simulink model "Converter_3"  (R2018a)
settings: Solver=ode45  StartTime=0.0  StopTime=3  RelTol=1e-3
InitFcn:
  | Ts=4e-4;
  | Ts_Power=Ts;
  | Ts_Control=Ts;
  | P_order = 0.9;
  | Q_order= 0.4;
  | V_order=1;
  | w_order = 1;
  | 
  | %outer loop
  | Kpvd=1;
  | Kivd=400;
  | Kpvq=1;
  | Kivq=10;
  | 
  | %inner loop
  | Kp=0.3;
  | Ki=5;
  | 
  | %Droop;
  | m=0.2;
  | n=0.1;
  | 
  | 
  | 
  | X=0.15;
  | wb=2*pi*60;
  | Sb=10e3; %2*Num MW
  | Vb=260;
  | Vconv=260;
  | Zb=Vb^2/Sb;
  | 
  | 
  | %% Tirp Transmision line
  | Tstep3=20; % trip line: Xg_start-->Xg_mid
  | Tstep2=30; % trip line: Xg_mid-->Xg_final
  | 
  | 
  | 
  | Xg_start=1.19; Xg_mid=1.2; Xg_final=1.21;
  | 
  | 
  | Xgpu2=Xg_mid*Xg_final/(Xg_final-Xg_mid);
  | Xgpu3=Xg_start*(Xg_final*Xgpu2)/(Xg_final*Xgpu2-Xg_start*(Xg_final+Xgpu2));
  | 
  | %Line 1
  | Xgpu1=Xg_final;
  | Rgpu1=0.1*Xgpu1;%Rg=0.1*Xg;
  | Xg1=Xgpu1*Zb;
  | Lg1=Xg1/wb;   %H
  | Rg1=Rgpu1*Zb; %ohm
  | %Line 2
  | Rgpu2=0.1*Xgpu2;%Rg=0.1*Xg;
  | Xg2=Xgpu2*Zb;
  | Lg2=Xg2/wb;   %H
  | Rg2=Rgpu2*Zb; %ohm
  | %Line 3
  | Rgpu3=0.1*Xgpu3;%Rg=0.1*Xg;
  | Xg3=Xgpu3*Zb;
  | Lg3=Xg3/wb;   %H
  | Rg3=Rgpu3*Zb; %ohm
undefined symbols (not defined in the file or in its folder): DiscIntNeverNeededParam
libraries: powerlib x14, simulink x3, powerlib_meascontrol x2, powerlib_extras x1
Description:
  | Copyright 2008-2018 The MathWorks, Inc.
settings Model: Creator=MathWorks  LastModifiedBy=almut
settings DataIOCC: FinalStateName=xFinal2  LimitDataPoints=on  SaveFinalState=on  SaveFormat=Array  SignalLoggingSaveFormat=ModelDataLogs
settings OptimizationCC: ExpressionDepthLimit=2147483647  LifeSpan=inf
settings DebuggingCC: AlgebraicLoopMsg=none  UnderspecifiedInitializationDetection=Classic  MergeDetectMultiDrivingBlocksExec=none  SolverPrmCheckMsg=warning  FcnCallInpInsideContextMsg=warning  StateNameClashWarn=warning  SFUnexpectedBacktrackingDiag=warning  SFNoUnconditionalDefaultTransitionDiag=warning  SFExecutionAtInitializationDiag=none
settings HardwareCC: ProdBitPerPointer=32  ProdBitPerSizeT=32  ProdBitPerPtrDiffT=32  ProdLargestAtomicFloat=None  ProdIntDivRoundTo=Undefined  ProdEndianess=Unspecified  ProdWordSize=32  ProdHWDeviceType=32-bit Generic
settings ModelReferenceCC: PropagateSignalLabelsOutOfModel=off
settings CodeAppCC: StateflowObjectComments=on
settings GRTTargetCC: TargetLangStandard=C89/C90 (ANSI)  GeneratePreprocessorConditionals=Disable all  CombineOutputUpdateFcns=off  GRTInterface=on
settings ConfigComp: CovMetricSettings=dw  CovHtmlReporting=on  CovSaveCumulativeToWorkspaceVar=on  CovSaveSingleToWorkspaceVar=on  CovExternalEMLEnable=off  CovSFcnEnable=off
settings SimscapeCC: SimscapeNormalizeSystem=off

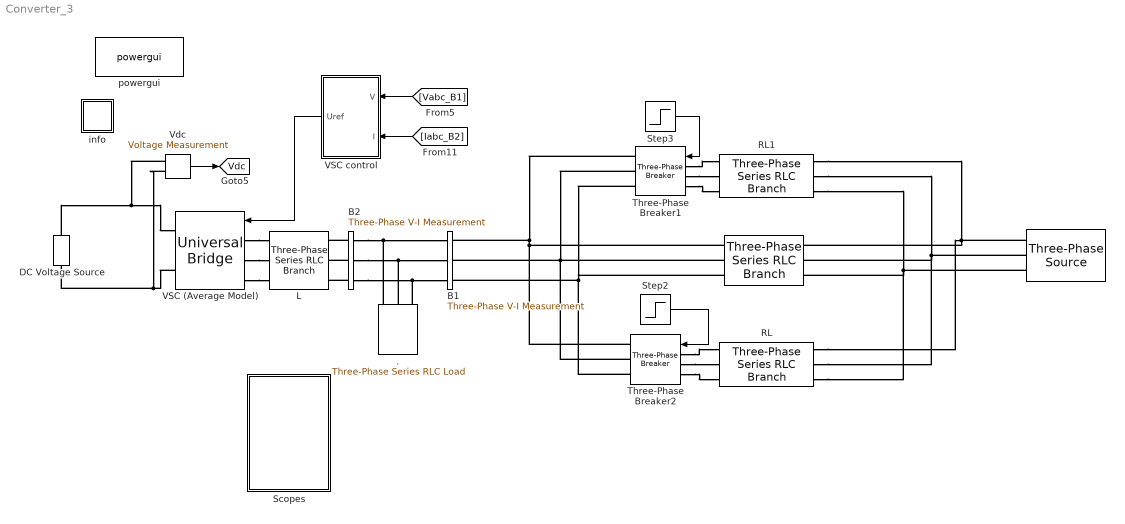
== system Converter_3 ==
  " " : powerlib/Elements/Three-Phase Series RLC Branch  LConnTagsString=A|B|C  RConnTagsString=A|B|C  BranchType=RL  Resistance=Rg1  Inductance=Lg1  Capacitance=[]  Measurements=None
  "   " : powerlib/Electrical Sources/Three-Phase Source  InternalConnection=Yg  VoltagePhases=off  Voltage=260  PhaseAngle=0  Voltage_phases=[25e3 25e3 25e3]/sqrt(3)  PhaseAngles_phases=[0 -120 +120]  Frequency=60  NonIdealSource=off  SpecifyImpedance=on  Resistance=0.8929  Inductance=16.58e-3  ShortCircuitLevel=2500e6  BaseVoltage=120e3  XRratio=7  BusType=swing  Pref=0  Qref=0  Prefabc=[10e3, 10e3, 10e3]  Qrefabc=[0, 0, 0]  Qmin=-inf  Qmax=inf
  "  ." : powerlib/Elements/Three-Phase Series RLC Load  LConnTagsString=A|B|C  Configuration=Y (grounded)  NominalVoltage=260  Vabc=[1e3 1e3 1e3]  Vabcp=[1e3 1e3 1e3]  NominalFrequency=60  UnbalancedPower=off  ActivePower=0  InductivePower=0  CapacitivePower=10e3*0.25  Pabc=[10e3 9e3 11e3]  QLabc=[100 90 110]  QCabc=[100 90 110]  Pabcp=[10e3 9e3 11e3]  QLabcp=[100 90 110]  QCabcp=[100 90 110]  Measurements=None  LoadType=constant Z
  B1 : powerlib/Measurements/Three-Phase V-I Measurement  VoltageMeasurement=phase-to-ground  SetLabelV=on  LabelV=Vabc_B1  Vpu=on  VpuLL=off  CurrentMeasurement=yes  SetLabelI=on  LabelI=Iabc_B1  Ipu=on  Pbase=10e3  Vbase=260  OutputType=Magnitude  PhasorSimulation=off  PSBequivalent=0
  B2 : powerlib/Measurements/Three-Phase V-I Measurement  VoltageMeasurement=phase-to-ground  SetLabelV=on  LabelV=Vabc_c  Vpu=on  VpuLL=off  CurrentMeasurement=yes  SetLabelI=on  LabelI=Iabc_B2  Ipu=on  Pbase=10e3  Vbase=260  OutputType=Magnitude  PhasorSimulation=off  PSBequivalent=0
  DC Voltage Source : powerlib/Electrical Sources/DC Voltage Source  Amplitude=500  Measurements=None
  L : powerlib/Elements/Three-Phase Series RLC Branch  LConnTagsString=A|B|C  RConnTagsString=A|B|C  BranchType=RL  Resistance=X/50*260^2/10e3  Inductance=X/(2*pi*60)*260^2/10e3  Capacitance=inf  Measurements=None
  RL : powerlib/Elements/Three-Phase Series RLC Branch  LConnTagsString=A|B|C  RConnTagsString=A|B|C  BranchType=RL  Resistance=Rg2  Inductance=Lg2  Capacitance=[]  Measurements=None
  RL1 : powerlib/Elements/Three-Phase Series RLC Branch  LConnTagsString=A|B|C  RConnTagsString=A|B|C  BranchType=RL  Resistance=Rg3  Inductance=Lg3  Capacitance=[]  Measurements=None
  Scopes : Subsystem
  Step2 : Step  Time=Tstep2  Before=1  After=0  SampleTime=0
  Step3 : Step  Time=Tstep3  Before=1  After=0  SampleTime=0
  Three-Phase Breaker1 : powerlib/Elements/Three-Phase Breaker  InitialState=closed  SwitchA=on  SwitchB=on  SwitchC=on  SwitchTimes=[1 1000]  External=on  BreakerResistance=0.001  SnubberResistance=1e6  SnubberCapacitance=inf  Measurements=None
  Three-Phase Breaker2 : powerlib/Elements/Three-Phase Breaker  InitialState=closed  SwitchA=on  SwitchB=on  SwitchC=on  SwitchTimes=[1 1000]  External=on  BreakerResistance=0.001  SnubberResistance=1e6  SnubberCapacitance=inf  Measurements=None
  VSC (Average Model) : powerlib/Power Electronics/Universal Bridge  Arms=3  SnubberResistance=1e5  SnubberCapacitance=inf  Device=Average-model based VSC  Ron=1e-3  Lon=0  ForwardVoltages="[  0  0  ]"  ForwardVoltage=0  GTOparameters=[ 10e-6 , 20e-6 ]  IGBTparameters=[ 1e-6 , 2e-6 ]  Measurements=None  Measurements_2=None  converterType=Rectifier
  VSC control : Subsystem
  "Vdc " : powerlib/Measurements/Voltage Measurement  Tag=PoWeRsYsTeMmEaSuReMeNt  PhasorSimulation=off  OutputType=Magnitude  PSBequivalent=0
  info : Subsystem
      settings: OpenFcn=showdemo(bdroot(gcb))
      mask Display: disp('?')
  powergui : powerlib/powergui  Priority=1  SimulationMode=Discrete  SampleTime=Ts_Power  frequency=60  Iterations=50  frequencyindice=0  Pbase=100e6  ErrMax=1e-4  UnitsV=kV  UnitsW=MW  buscounter=0  FunctionMessages=off  echomessages=off  EnableUseOfTLC=off  CurrentSourceSwitches=off  DisableSnubberDevices=off  DisableRonSwitches=off  DisableVfSwitches=off  DisplayEquations=off  SolverType=Tustin/Backward Euler (TBE)  Interpol=off  ExternalGateDelay=off  methode=off  Ts=100  x0status=blocks  SPID=off  SwTol=0  HookPort=off  RestoreLinks=warning  ResistiveCurrentMeasurement=off  Frange=[0:2:500]  Ylog=off  Xlog=on  ShowGrid=off  save=off  variable=ZData  structure=y1  ZoomFFT=off  StartTime=3  cycles=60  DisplayStyle=2  fundamental=60  FreqAxis=off  MaxFrequency=100  frequencyindicesteady=1  RmsSteady=1  display=off
  tag scope: Vdc=global
  wires:
  "Vdc "/1 -> [Vdc]
  [Vabc_B1] -> VSC control/1(V)
  [Iabc_B2] -> VSC control/2(I)
  VSC control/1(Uref) -> VSC (Average Model)/1
  Step2/1 -> Three-Phase Breaker2/1
  Step3/1 -> Three-Phase Breaker1/1
  connections:
  VSC (Average Model)/LConn1 -- L/LConn1
  VSC (Average Model)/LConn2 -- L/LConn2
  VSC (Average Model)/LConn3 -- L/LConn3
  B2/RConn3 -- "  ."/LConn3 -- B1/LConn3
  B2/RConn1 -- "  ."/LConn1 -- B1/LConn1
  B2/RConn2 -- "  ."/LConn2 -- B1/LConn2
  B2/LConn1 -- L/RConn1
  B2/LConn2 -- L/RConn2
  B2/LConn3 -- L/RConn3
  VSC (Average Model)/RConn2 -- "Vdc "/LConn2 -- DC Voltage Source/LConn1
  DC Voltage Source/RConn1 -- "Vdc "/LConn1 -- VSC (Average Model)/RConn1
  Three-Phase Breaker1/LConn2 -- RL1/RConn2
  Three-Phase Breaker1/LConn1 -- RL1/RConn1
  Three-Phase Breaker2/LConn2 -- RL/RConn2
  Three-Phase Breaker2/LConn1 -- RL/RConn1
  Three-Phase Breaker1/LConn3 -- RL1/RConn3
  Three-Phase Breaker2/LConn3 -- RL/RConn3
  Three-Phase Breaker2/RConn1 -- " "/RConn1 -- Three-Phase Breaker1/RConn1 -- B1/RConn1
  Three-Phase Breaker2/RConn2 -- " "/RConn2 -- Three-Phase Breaker1/RConn2 -- B1/RConn2
  Three-Phase Breaker2/RConn3 -- " "/RConn3 -- Three-Phase Breaker1/RConn3 -- B1/RConn3
  "   "/RConn1 -- RL/LConn1 -- " "/LConn1 -- RL1/LConn1
  "   "/RConn2 -- RL/LConn2 -- " "/LConn2 -- RL1/LConn2
  "   "/RConn3 -- RL/LConn3 -- " "/LConn3 -- RL1/LConn3

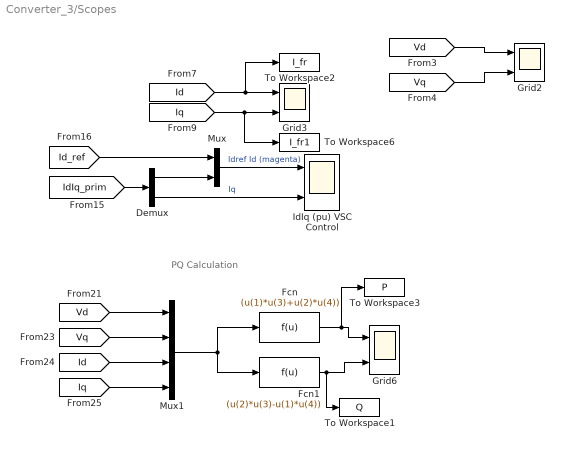
== system Converter_3/Scopes ==
  note: PQ Calculation
  Demux : Demux  Outputs=2
  Fcn : Fcn  Expr=(u(1)*u(3)+u(2)*u(4))
  Fcn1 : Fcn  Expr=(u(2)*u(3)-u(1)*u(4))
  Grid2 : Scope  NumInputPorts=2
  Grid3 : Scope  NumInputPorts=2
  Grid6 : Scope  NumInputPorts=2
  IdIq (pu) VSC Control : Scope  NumInputPorts=2
  Mux : Mux  Inputs=2
  Mux1 : Mux
  To Workspace1 : ToWorkspace  VariableName=Q  SaveFormat=Timeseries  SampleTime=Ts
      settings: Save2DSignal=2-D array (concatenate along first dimension)
  To Workspace2 : ToWorkspace  VariableName=I_fr  SaveFormat=Timeseries  SampleTime=Ts
      settings: Save2DSignal=2-D array (concatenate along first dimension)
  To Workspace3 : ToWorkspace  VariableName=P  SaveFormat=Timeseries  SampleTime=Ts
      settings: Save2DSignal=2-D array (concatenate along first dimension)
  To Workspace6 : ToWorkspace  VariableName=I_fr1  SaveFormat=Timeseries  SampleTime=Ts
      settings: Save2DSignal=2-D array (concatenate along first dimension)
  wires:
  [Id] -> To Workspace2/1, Grid3/1
  Mux/1 -> IdIq (pu) VSC Control/1  "Idref Id (magenta)"
  Demux/2 -> IdIq (pu) VSC Control/2  "Iq"
  [Vq] -> Grid2/2
  [Id_ref] -> Mux/1
  Demux/1 -> Mux/2
  [Iq] -> To Workspace6/1, Grid3/2
  [Vd] -> Grid2/1
  [IdIq_prim] -> Demux/1
  [Vd] -> Mux1/1
  [Id] -> Mux1/3
  Fcn/1 -> To Workspace3/1, Grid6/1
  [Vq] -> Mux1/2
  [Iq] -> Mux1/4
  Mux1/1 -> Fcn/1, Fcn1/1
  Fcn1/1 -> To Workspace1/1, Grid6/2

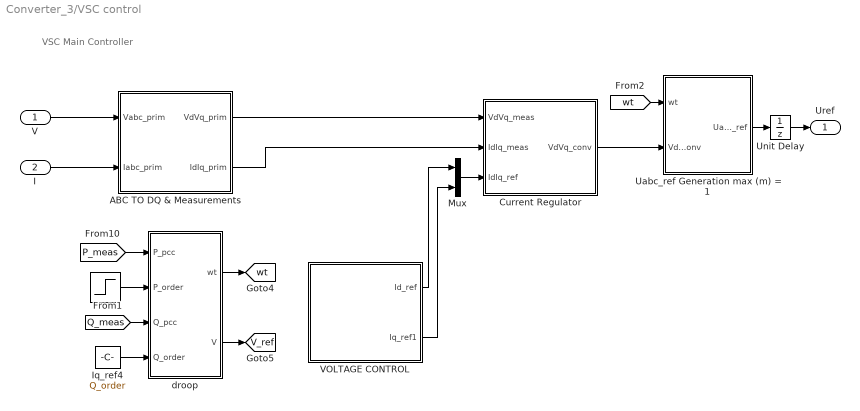
== system Converter_3/VSC control ==
  note: VSC Main Controller
  V : Inport  PortDimensions=3
  I : Inport  Port=2  PortDimensions=3
  " " : Step  Time=2  Before=P_order  After=0.91  SampleTime=0
  ABC TO DQ & Measurements : Subsystem
  Current Regulator : Subsystem
  Iq_ref4 : Constant  Value=Q_order
  Mux : Mux  Inputs=2
  Uabc_ref Generation max (m) = 1 : Subsystem
  Unit Delay : UnitDelay  SampleTime=Ts_Control
  VOLTAGE CONTROL : Subsystem
  droop : Subsystem
  Uref : Outport
  tag scope: V_ref=global, wt=global
  wires:
  Iq_ref4/1 -> droop/4(Q_order)
  " "/1 -> droop/2(P_order)
  [P_meas] -> droop/1(P_pcc)
  [Q_meas] -> droop/3(Q_pcc)
  droop/1(wt) -> [wt]
  droop/2(V) -> [V_ref]
  Current Regulator/1(VdVq_conv) -> Uabc_ref Generation max (m) = 1/2(VdVq_conv)
  ABC TO DQ & Measurements/2(IdIq_prim) -> Current Regulator/2(IdIq_meas)
  VOLTAGE CONTROL/1(Id_ref) -> Mux/1
  ABC TO DQ & Measurements/1(VdVq_prim) -> Current Regulator/1(VdVq_meas)
  Unit Delay/1 -> Uref/1
  [wt] -> Uabc_ref Generation max (m) = 1/1(wt)
  V/1 -> ABC TO DQ & Measurements/1(Vabc_prim)
  I/1 -> ABC TO DQ & Measurements/2(Iabc_prim)
  VOLTAGE CONTROL/2(Iq_ref1) -> Mux/2
  Uabc_ref Generation max (m) = 1/1(Uabc_ref) -> Unit Delay/1
  Mux/1 -> Current Regulator/3(IdIq_ref)

== system Converter_3/info ==

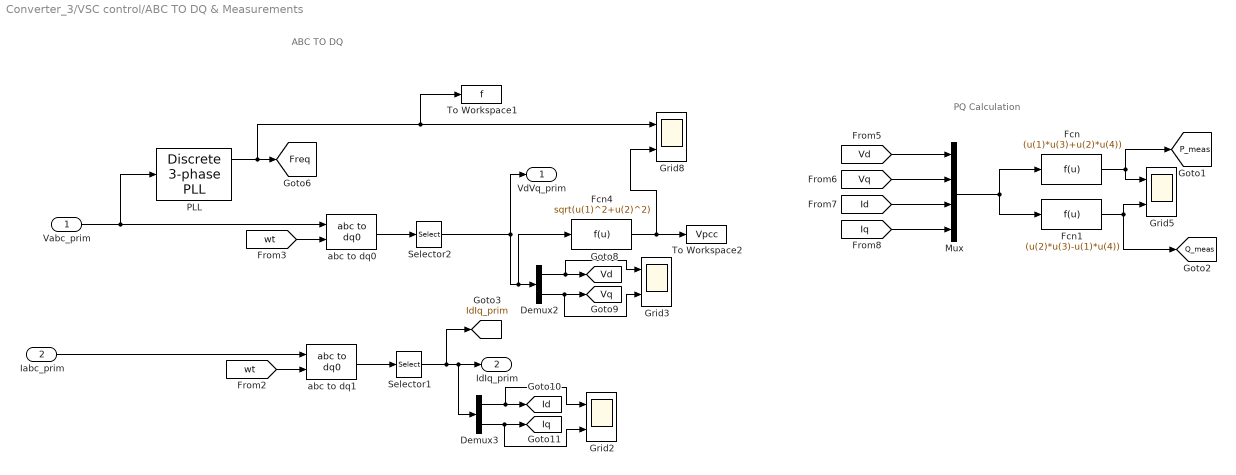
== system Converter_3/VSC control/ABC TO DQ & Measurements ==
  note: PQ Calculation
  note: ABC TO DQ
  Vabc_prim : Inport
  Iabc_prim : Inport  Port=2
  Demux2 : Demux  Outputs=2
  Demux3 : Demux  Outputs=2
  Fcn : Fcn  Expr=(u(1)*u(3)+u(2)*u(4))
  Fcn1 : Fcn  Expr=(u(2)*u(3)-u(1)*u(4))
  Fcn4 : Fcn  Expr=sqrt(u(1)^2+u(2)^2)
  Grid{2..3,5,8} (4 alike) : Scope  NumInputPorts=2
  Mux : Mux
  PLL : powerlib_extras/Discrete  Control Blocks/Discrete 3-phase PLL  Fmin=45  Par_Init="[-0.57  60]"  ParK=[60 1400]  Ts=Ts  AGC=off
  Selector1 : Selector  InputPortWidth=3  IndexOptions=Index vector (dialog)  Indices=[1 2]  OutputSizes=1
  Selector2 : Selector  InputPortWidth=3  IndexOptions=Index vector (dialog)  Indices=[1 2]  OutputSizes=1
  To Workspace1 : ToWorkspace  VariableName=f  SaveFormat=Timeseries  SampleTime=Ts
      settings: Save2DSignal=2-D array (concatenate along first dimension)
  To Workspace2 : ToWorkspace  VariableName=Vpcc  SaveFormat=Timeseries  SampleTime=Ts
      settings: Save2DSignal=2-D array (concatenate along first dimension)
  abc to dq0 : powerlib_meascontrol/Transformations/abc to dq0  Alignment=90 degrees behind phase A axis
  abc to dq1 : powerlib_meascontrol/Transformations/abc to dq0  Alignment=90 degrees behind phase A axis
  VdVq_prim : Outport
  IdIq_prim : Outport  Port=2
  tag scope: Freq=global, Id=global, IdIq_prim=global, Iq=global, P_meas=global, Q_meas=global, Vd=global, Vq=global
  wires:
  Selector2/1 -> Fcn4/1, Demux2/1, VdVq_prim/1
  abc to dq0/1 -> Selector2/1
  abc to dq1/1 -> Selector1/1
  Vabc_prim/1 -> PLL/1, abc to dq0/1
  Iabc_prim/1 -> abc to dq1/1
  Demux2/2 -> Grid3/2, [Vq]
  Demux3/1 -> [Id], Grid2/1
  Demux3/2 -> Grid2/2, [Iq]
  [wt] -> abc to dq0/2
  [wt] -> abc to dq1/2
  Selector1/1 -> Demux3/1, IdIq_prim/1, [IdIq_prim]
  PLL/1 -> To Workspace1/1, Grid8/1, [Freq]
  Demux2/1 -> Grid3/1, [Vd]
  [Vd] -> Mux/1
  [Id] -> Mux/3
  [Iq] -> Mux/4
  Mux/1 -> Fcn/1, Fcn1/1
  Fcn/1 -> [P_meas], Grid5/1
  Fcn1/1 -> [Q_meas], Grid5/2
  [Vq] -> Mux/2
  Fcn4/1 -> To Workspace2/1, Grid8/2

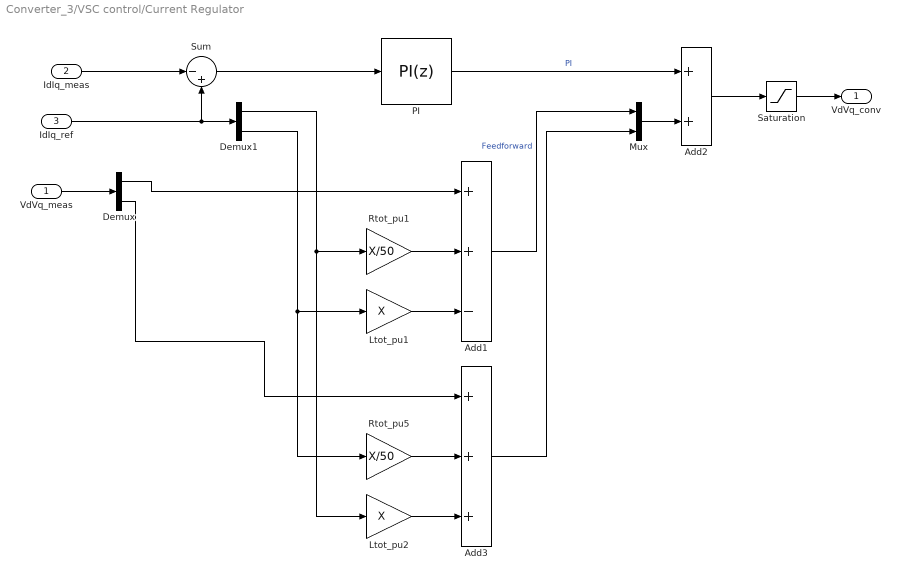
== system Converter_3/VSC control/Current Regulator ==
  VdVq_meas : Inport  PortDimensions=2
  IdIq_meas : Inport  Port=2  PortDimensions=2
  IdIq_ref : Inport  Port=3  PortDimensions=2
  Add1 : Sum  Inputs=++-
  Add2 : Sum
  Add3 : Sum  Inputs=+++
  Demux : Demux  Outputs=2
  Demux1 : Demux  Outputs=2
  Ltot_pu1 : Gain  Gain=X  SaturateOnIntegerOverflow=on  OutDataTypeStr=Inherit: Same as input  ParamDataTypeStr=Inherit: Same as input
  Ltot_pu2 : Gain  Gain=X  SaturateOnIntegerOverflow=on  OutDataTypeStr=Inherit: Same as input  ParamDataTypeStr=Inherit: Same as input
  Mux : Mux  Inputs=2
  PI : simulink/Continuous/PID Controller  Controller=PI  TimeDomain=Discrete-time  SampleTime=Ts  IntegratorMethod=Forward Euler  FilterMethod=Forward Euler  Form=Parallel  UseFilter=on  ControllerParametersSource=internal  P=Kp  I=Ki  D=0  N=100  InitialConditionSource=internal  InitialConditionForIntegrator=0  InitialConditionForFilter=0  ExternalReset=none  LimitOutput=on  UpperSaturationLimit=2  LowerSaturationLimit=-2  LinearizeAsGain=off  AntiWindupMode=none  Kb=1  TrackingMode=off  Kt=1  PParamMin=[]  PParamMax=[]  IParamMin=[]  IParamMax=[]  DParamMin=[]  DParamMax=[]  NParamMin=[]  NParamMax=[]  KbParamMin=[]  KbParamMax=[]  KtParamMin=[]  KtParamMax=[]  POutMin=[]  POutMax=[]  IOutMin=[]  IOutMax=[]  DOutMin=[]  DOutMax=[]  NOutMin=[]  NOutMax=[]  KbOutMin=[]  KbOutMax=[]  KtOutMin=[]  KtOutMax=[]  IntegratorOutMin=[]  IntegratorOutMax=[]  FilterOutMin=[]  FilterOutMax=[]  SumOutMin=[]  SumOutMax=[]  SumI1OutMin=[]  SumI1OutMax=[]  SumI2OutMin=[]  SumI2OutMax=[]  SumI3OutMin=[]  SumI3OutMax=[]  SumDOutMin=[]  SumDOutMax=[]  SaturationOutMin=[]  SaturationOutMax=[]  IntegratorContinuousStateAttributes=''  IntegratorStateMustResolveToSignalObject=off  IntegratorRTWStateStorageClass=Auto  FilterContinuousStateAttributes=''  FilterStateMustResolveToSignalObject=off  FilterRTWStateStorageClass=Auto  DifferentiatorICPrevScaledInput=0  DifferentiatorOutMin=[]  DifferentiatorOutMax=[]  FilterDiffOutCoefMin=[]  FilterDiffOutCoefMax=[]  SumDenOutMin=[]  SumDenOutMax=[]  SumNumOutMin=[]  SumNumOutMax=[]  ReciprocalOutMin=[]  ReciprocalOutMax=[]  DivideOutMin=[]  DivideOutMax=[]  TunerSelectOption=Transfer Function Based (PID Tuner App)
  Rtot_pu1 : Gain  Gain=X/50  SaturateOnIntegerOverflow=on  OutDataTypeStr=Inherit: Same as input  ParamDataTypeStr=Inherit: Same as input
  Rtot_pu5 : Gain  Gain=X/50  SaturateOnIntegerOverflow=on  OutDataTypeStr=Inherit: Same as input  ParamDataTypeStr=Inherit: Same as input
  Saturation : Saturate  UpperLimit=2  LowerLimit=-2
  Sum : Sum  Inputs=|-+
  VdVq_conv : Outport
  wires:
  Add3/1 -> Mux/2
  Add1/1 -> Mux/1  "Feedforward"
  Ltot_pu2/1 -> Add3/3
  Rtot_pu5/1 -> Add3/2
  Demux1/2 -> Rtot_pu5/1, Ltot_pu1/1
  Ltot_pu1/1 -> Add1/3
  Demux1/1 -> Ltot_pu2/1, Rtot_pu1/1
  Rtot_pu1/1 -> Add1/2
  VdVq_meas/1 -> Demux/1
  Saturation/1 -> VdVq_conv/1
  Add2/1 -> Saturation/1
  IdIq_meas/1 -> Sum/1
  IdIq_ref/1 -> Demux1/1, Sum/2
  Sum/1 -> PI/1
  PI/1 -> Add2/1  "PI"
  Mux/1 -> Add2/2
  Demux/1 -> Add1/1
  Demux/2 -> Add3/1

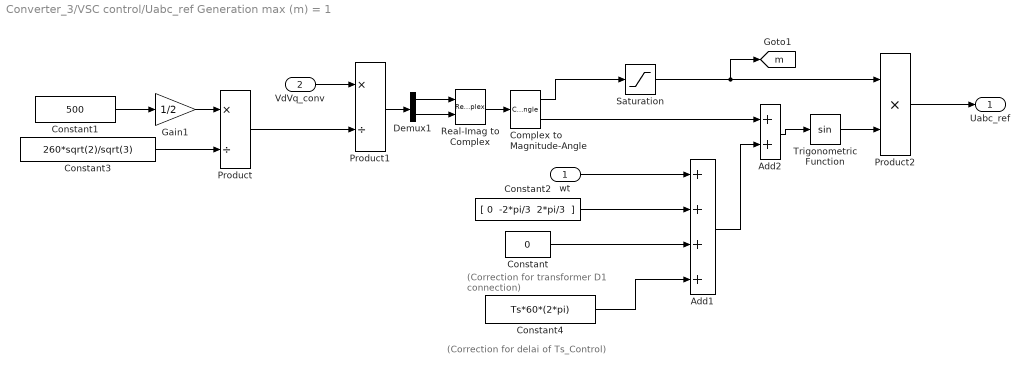
== system Converter_3/VSC control/Uabc_ref Generation max (m) = 1 ==
  note: (Correction for delai of Ts_Control)
  note: (Correction for transformer
      |  D1 connection)
  wt : Inport
  VdVq_conv : Inport  Port=2
  Add1 : Sum  Inputs=++++
  Add2 : Sum
  Complex to Magnitude-Angle : ComplexToMagnitudeAngle
  Constant : Constant  Value=0
  Constant1 : Constant  Value=500
  Constant2 : Constant  Value="[ 0  -2*pi/3  2*pi/3  ]"
  Constant3 : Constant  Value=260*sqrt(2)/sqrt(3)
  Constant4 : Constant  Value=Ts*60*(2*pi)
  Demux1 : Demux  Outputs=2
  Gain1 : Gain  Gain=1/2
  Product : Product  Inputs=*/  RndMeth=Zero
  Product1 : Product  Inputs=*/  RndMeth=Zero
  Product2 : Product  Inputs=**  RndMeth=Zero
  Real-Imag to Complex : RealImagToComplex
  Saturation : Saturate  UpperLimit=0.95  LowerLimit=0
  Trigonometric Function : Trigonometry
  Uabc_ref : Outport
  tag scope: m=global
  wires:
  Constant4/1 -> Add1/4
  wt/1 -> Add1/1
  Product2/1 -> Uabc_ref/1
  Trigonometric Function/1 -> Product2/2
  Saturation/1 -> Product2/1, [m]
  Add2/1 -> Trigonometric Function/1
  Add1/1 -> Add2/2
  Complex to Magnitude-Angle/2 -> Add2/1
  Product/1 -> Product1/2
  Constant3/1 -> Product/2
  Constant/1 -> Add1/3
  Constant2/1 -> Add1/2
  Demux1/2 -> Real-Imag to Complex/2
  Demux1/1 -> Real-Imag to Complex/1
  Real-Imag to Complex/1 -> Complex to Magnitude-Angle/1
  Gain1/1 -> Product/1
  Product1/1 -> Demux1/1
  VdVq_conv/1 -> Product1/1
  Constant1/1 -> Gain1/1
  Complex to Magnitude-Angle/1 -> Saturation/1

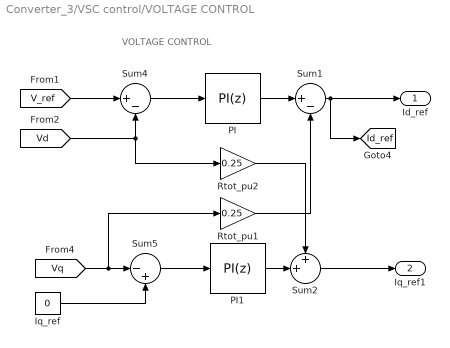
== system Converter_3/VSC control/VOLTAGE CONTROL ==
  note: VOLTAGE CONTROL
  Iq_ref : Constant  Value=0
  PI : simulink/Continuous/PID Controller  Controller=PI  TimeDomain=Discrete-time  SampleTime=Ts  IntegratorMethod=Trapezoidal  FilterMethod=Forward Euler  Form=Parallel  UseFilter=on  ControllerParametersSource=internal  P=Kpvd  I=Kivd  D=0  N=100  InitialConditionSource=internal  InitialConditionForIntegrator=0  InitialConditionForFilter=0  ExternalReset=none  LimitOutput=on  UpperSaturationLimit=1.5  LowerSaturationLimit=-1.5  LinearizeAsGain=off  AntiWindupMode=none  Kb=1  TrackingMode=off  Kt=1  PParamMin=[]  PParamMax=[]  IParamMin=[]  IParamMax=[]  DParamMin=[]  DParamMax=[]  NParamMin=[]  NParamMax=[]  KbParamMin=[]  KbParamMax=[]  KtParamMin=[]  KtParamMax=[]  POutMin=[]  POutMax=[]  IOutMin=[]  IOutMax=[]  DOutMin=[]  DOutMax=[]  NOutMin=[]  NOutMax=[]  KbOutMin=[]  KbOutMax=[]  KtOutMin=[]  KtOutMax=[]  IntegratorOutMin=[]  IntegratorOutMax=[]  FilterOutMin=[]  FilterOutMax=[]  SumOutMin=[]  SumOutMax=[]  SumI1OutMin=[]  SumI1OutMax=[]  SumI2OutMin=[]  SumI2OutMax=[]  SumI3OutMin=[]  SumI3OutMax=[]  SumDOutMin=[]  SumDOutMax=[]  SaturationOutMin=[]  SaturationOutMax=[]  IntegratorContinuousStateAttributes=''  IntegratorStateMustResolveToSignalObject=off  IntegratorRTWStateStorageClass=Auto  FilterContinuousStateAttributes=''  FilterStateMustResolveToSignalObject=off  FilterRTWStateStorageClass=Auto  DifferentiatorICPrevScaledInput=0  DifferentiatorOutMin=[]  DifferentiatorOutMax=[]  FilterDiffOutCoefMin=[]  FilterDiffOutCoefMax=[]  SumDenOutMin=[]  SumDenOutMax=[]  SumNumOutMin=[]  SumNumOutMax=[]  ReciprocalOutMin=[]  ReciprocalOutMax=[]  DivideOutMin=[]  DivideOutMax=[]  TunerSelectOption=Transfer Function Based (PID Tuner App)
  PI1 : simulink/Continuous/PID Controller  Controller=PI  TimeDomain=Discrete-time  SampleTime=Ts  IntegratorMethod=Trapezoidal  FilterMethod=Forward Euler  Form=Parallel  UseFilter=on  ControllerParametersSource=internal  P=Kpvq  I=Kivq  D=0  N=100  InitialConditionSource=internal  InitialConditionForIntegrator=0  InitialConditionForFilter=0  ExternalReset=none  LimitOutput=on  UpperSaturationLimit=1.5  LowerSaturationLimit=-1.05  LinearizeAsGain=off  AntiWindupMode=none  Kb=1  TrackingMode=off  Kt=1  PParamMin=[]  PParamMax=[]  IParamMin=[]  IParamMax=[]  DParamMin=[]  DParamMax=[]  NParamMin=[]  NParamMax=[]  KbParamMin=[]  KbParamMax=[]  KtParamMin=[]  KtParamMax=[]  POutMin=[]  POutMax=[]  IOutMin=[]  IOutMax=[]  DOutMin=[]  DOutMax=[]  NOutMin=[]  NOutMax=[]  KbOutMin=[]  KbOutMax=[]  KtOutMin=[]  KtOutMax=[]  IntegratorOutMin=[]  IntegratorOutMax=[]  FilterOutMin=[]  FilterOutMax=[]  SumOutMin=[]  SumOutMax=[]  SumI1OutMin=[]  SumI1OutMax=[]  SumI2OutMin=[]  SumI2OutMax=[]  SumI3OutMin=[]  SumI3OutMax=[]  SumDOutMin=[]  SumDOutMax=[]  SaturationOutMin=[]  SaturationOutMax=[]  IntegratorContinuousStateAttributes=''  IntegratorStateMustResolveToSignalObject=off  IntegratorRTWStateStorageClass=Auto  FilterContinuousStateAttributes=''  FilterStateMustResolveToSignalObject=off  FilterRTWStateStorageClass=Auto  DifferentiatorICPrevScaledInput=0  DifferentiatorOutMin=[]  DifferentiatorOutMax=[]  FilterDiffOutCoefMin=[]  FilterDiffOutCoefMax=[]  SumDenOutMin=[]  SumDenOutMax=[]  SumNumOutMin=[]  SumNumOutMax=[]  ReciprocalOutMin=[]  ReciprocalOutMax=[]  DivideOutMin=[]  DivideOutMax=[]  TunerSelectOption=Transfer Function Based (PID Tuner App)
  Rtot_pu1 : Gain  Gain=0.25  SaturateOnIntegerOverflow=on  OutDataTypeStr=Inherit: Same as input  ParamDataTypeStr=Inherit: Same as input
  Rtot_pu2 : Gain  Gain=0.25  SaturateOnIntegerOverflow=on  OutDataTypeStr=Inherit: Same as input  ParamDataTypeStr=Inherit: Same as input
  Sum1 : Sum  Inputs=|+-
  Sum2 : Sum  Inputs=++|
  Sum4 : Sum  Inputs=|+-
  Sum5 : Sum  Inputs=|-+
  Id_ref : Outport  SampleTime=Ts  InitialOutput=0
  Iq_ref1 : Outport  Port=2  SampleTime=Ts  InitialOutput=0
  tag scope: Id_ref=global
  wires:
  Sum4/1 -> PI/1
  Sum5/1 -> PI1/1
  Iq_ref/1 -> Sum5/2
  Rtot_pu1/1 -> Sum1/2
  PI1/1 -> Sum2/2
  Rtot_pu2/1 -> Sum2/1
  Sum1/1 -> [Id_ref], Id_ref/1
  Sum2/1 -> Iq_ref1/1
  PI/1 -> Sum1/1
  [Vq] -> Rtot_pu1/1, Sum5/1
  [V_ref] -> Sum4/1
  [Vd] -> Rtot_pu2/1, Sum4/2

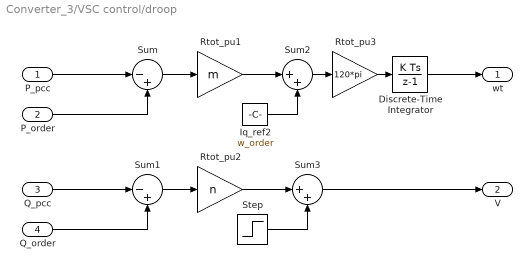
== system Converter_3/VSC control/droop ==
  P_pcc : Inport
  P_order : Inport  Port=2
  Q_pcc : Inport  Port=3
  Q_order : Inport  Port=4
  Discrete-Time Integrator : DiscreteIntegrator  SampleTime=Ts  ICPrevOutput=DiscIntNeverNeededParam  ICPrevScaledInput=DiscIntNeverNeededParam
  Iq_ref2 : Constant  Value=w_order
  Rtot_pu1 : Gain  Gain=m  SaturateOnIntegerOverflow=on  OutDataTypeStr=Inherit: Same as input  ParamDataTypeStr=Inherit: Same as input
  Rtot_pu2 : Gain  Gain=n  SaturateOnIntegerOverflow=on  OutDataTypeStr=Inherit: Same as input  ParamDataTypeStr=Inherit: Same as input
  Rtot_pu3 : Gain  Gain=120*pi  SaturateOnIntegerOverflow=on  OutDataTypeStr=Inherit: Same as input  ParamDataTypeStr=Inherit: Same as input
  Step : Step  Time=33  Before=V_order  After=1.06  SampleTime=0
  Sum : Sum  Inputs=|-+
  Sum1 : Sum  Inputs=|-+
  Sum2 : Sum  Inputs=|++
  Sum3 : Sum  Inputs=|++
  wt : Outport
  V : Outport  Port=2
  wires:
  Step/1 -> Sum3/2
  Sum2/1 -> Rtot_pu3/1
  Sum/1 -> Rtot_pu1/1
  Sum1/1 -> Rtot_pu2/1
  Discrete-Time Integrator/1 -> wt/1
  Rtot_pu2/1 -> Sum3/1
  Rtot_pu3/1 -> Discrete-Time Integrator/1
  Rtot_pu1/1 -> Sum2/1
  Iq_ref2/1 -> Sum2/2
  P_pcc/1 -> Sum/1
  Sum3/1 -> V/1
  Q_order/1 -> Sum1/2
  P_order/1 -> Sum/2
  Q_pcc/1 -> Sum1/1
